simulink model "fft_magnitude"  (R2018a)
settings: Solver=VariableStepAuto  StartTime=0.0  StopTime=10.0  RelTol=1e-3
libraries: dspmathops x1
settings Model: Creator=berke  LastModifiedBy=berke

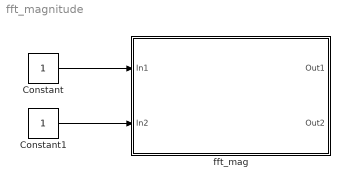
== system fft_magnitude ==
  Constant : Constant  OutDataTypeStr=fixdt(1,13,12)  SampleTime=0.1
  Constant1 : Constant  OutDataTypeStr=boolean  SampleTime=0.1
  fft_mag : Subsystem
  wires:
  Constant/1 -> fft_mag/1(In1)
  Constant1/1 -> fft_mag/2(In2)

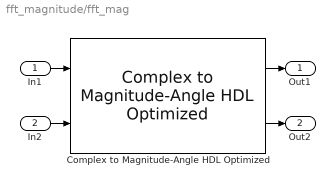
== system fft_magnitude/fft_mag ==
  In1 : Inport
  In2 : Inport  Port=2
  Complex to Magnitude-Angle HDL Optimized : dspmathops/Complex to Magnitude-Angle HDL Optimized  NumIterationsSource=Auto  NumIterations=10  OutputFormat=Magnitude  AngleFormat=Normalized  ScaleOutput=on  SimulateUsing=Code generation
      settings: SourceProductName=DSP System Toolbox  SourceProductBaseCode=DS
  Out1 : Outport
  Out2 : Outport  Port=2
  wires:
  In2/1 -> Complex to Magnitude-Angle HDL Optimized/2
  In1/1 -> Complex to Magnitude-Angle HDL Optimized/1
  Complex to Magnitude-Angle HDL Optimized/1 -> Out1/1
  Complex to Magnitude-Angle HDL Optimized/2 -> Out2/1
